simulink subsystem "Day6_Scenario_1"  (R2024a)
settings: Solver=VariableStepAuto  StartTime=0.0  StopTime=10.0  RelTol=1e-3
undefined symbols (not defined in the file): DiscIntNeverNeededParam, route1_waypoint, route2_waypoint, route3_waypoint
libraries: CarMaker4SL x42, simulink x1
(part 2 of 2)

== matlab function Day6_Scenario_1/MATLAB Function19 ==
  settings: sampleTime=0.1
  data: ego_pos input; ego_yaw input; ego_vx input; target_speed input; route1_waypoint input; FrontTireAngle output; DesiredAx output; x_local output; y_local output; lane_id_out output; route2_waypoint input; route3_waypoint input; dt input
% function [FrontTireAngle, DesiredAx, x_local, y_local, lane_id_out] = lane_follower_allin1( ...
%     ego_pos, ego_yaw, ego_vx, target_speed, ...
%     route1_waypoint, route2_waypoint, route3_waypoint, dt)
% % 하나의 블록에서 10초마다 차선 바꾸면서 해당 차선 추종
% 
% %% 1. 10초 주기 lane_id 변경 (시퀀스)
% persistent elapsed lane_idx
% seq = [1 2 3 2 1 2]; % 순환 패턴
% Nseq = length(seq);
% T = 15; % 10초
% 
% if isempty(elapsed)
%     elapsed = 0;
%     lane_idx = 1;
% end
% 
% elapsed = elapsed + dt;
% if elapsed >= T
%     lane_idx = mod(lane_idx, Nseq) + 1;
%     elapsed = 0;
% end
% lane_id = seq(lane_idx);
% lane_id_out = lane_id; % (디버깅/Scope 출력용)
% 
% %% 2. 차선별 route 선택
% if lane_id == 1
%     waypoints = route1_waypoint;
% elseif lane_id == 2
%     waypoints = route2_waypoint;
% elseif lane_id == 3
%     waypoints = route3_waypoint;
% else
%     waypoints = route1_waypoint; % 예외
% end
% 
% %% 3. 이하 기존 웨이포인트 추종 로직 (필요시 복사/수정)
% ego_x = ego_pos(1);
% ego_y = ego_pos(2);
% 
% % 샘플링
% sample_gap = 10;
% x = waypoints(1:sample_gap:end,1);
% y = waypoints(1:sample_gap:end,2);
% 
% % 이상치 필터링
% dx = diff(x); dy = diff(y);
% d = sqrt(dx.^2 + dy.^2);
% thresh = mean(d) + 4*std(d);
% normal_idx = find([true; d < thresh]);
% x_filt = x(normal_idx);
% y_filt = y(normal_idx);
% 
% % 폐곡선 보장
% if norm([x_filt(1), y_filt(1)] - [x_filt(end), y_filt(end)]) > 1e-3
%     x_filt = [x_filt; x_filt(1)];
%     y_filt = [y_filt; y_filt(1)];
% end
% 
% N = length(x_filt);
% 
% % 보간
% interp_ratio = 3;
% max_interp = min(10000, interp_ratio*N);
% t = (1:N)';
% tq = linspace(1, N, max_interp)';
% route_xq = interp1(t, x_filt, tq, 'spline');
% route_yq = interp1(t, y_filt, tq, 'spline');
% Nq = length(route_xq);
% 
% % 윈도우/인덱스 관리
% persistent prev_idx
% if isempty(prev_idx)
%     dist_init = sqrt((route_xq - ego_x).^2 + (route_yq - ego_y).^2);
%     [~, prev_idx] = min(dist_init);
% end
% 
% window_size = 300;
% idx_win = mod((prev_idx-window_size):(prev_idx+window_size)-1, Nq) + 1;
% 
% dx_win = route_xq(idx_win) - ego_x;
% dy_win = route_yq(idx_win) - ego_y;
% x_local_win = dx_win * cos(-ego_yaw) - dy_win * sin(-ego_yaw);
% y_local_win = dx_win * sin(-ego_yaw) + dy_win * cos(-ego_yaw);
% 
% % 진행방향(dot product) 기반 추종점 선택
% Nw = length(idx_win);
% tangent_vecs = zeros(Nw,2);
% for i=1:Nw
%     ip1 = mod(idx_win(i), Nq) + 1;
%     tangent_vecs(i,1) = route_xq(ip1) - route_xq(idx_win(i));
%     tangent_vecs(i,2) = route_yq(ip1) - route_yq(idx_win(i));
% end
% tangent_norm = sqrt(sum(tangent_vecs.^2,2));
% tangent_vecs = tangent_vecs ./ max(tangent_norm, 1e-6);
% 
% ego_heading = [cos(ego_yaw), sin(ego_yaw)];
% dotval = tangent_vecs * ego_heading';
% 
% valid_idx = find(x_local_win > 0 & dotval > 0.0);
% 
% if isempty(valid_idx)
%     [~, idx_sub] = min(sqrt(dx_win.^2 + dy_win.^2));
%     idx_min = idx_win(idx_sub);
%     idx_local = idx_sub;
% else
%     [~, idx_sub] = min(x_local_win(valid_idx).^2 + y_local_win(valid_idx).^2);
%     idx_min = idx_win(valid_idx(idx_sub));
%     idx_local = valid_idx(idx_sub);
% end
% 
% x_local = x_local_win(idx_local);
% y_local = y_local_win(idx_local);
% cte = y_local;
% prev_idx = mod(idx_min - 1, Nq) + 1;
% 
% % 횡방향 PD 제어 (조향)
% persistent prev_e prev_steer
% if isempty(prev_e)
%     prev_e = 0;
% end
% if isempty(prev_steer)
%     prev_steer = 0;
% end
% Kp = 0.2;   
% Kd = 0.01;
% d_e = (cte - prev_e) / dt;
% raw_steer = (Kp * cte + Kd * d_e);
% prev_e = cte;
% 
% % ====== 조향각 제한 ======
% STEER_LIMIT = 1; % [rad], ±28도 정도
% raw_steer = max(min(raw_steer, STEER_LIMIT), -STEER_LIMIT);
% 
% % ====== 조향각 변화율 제한 추가 ======
% MAX_STEER_RATE = 0.03;  % [rad/step] (예: 0.02rad/0.001s → 20rad/s)
% delta_steer = raw_steer - prev_steer;
% delta_steer = max(min(delta_steer, MAX_STEER_RATE), -MAX_STEER_RATE);
% 
% FrontTireAngle = prev_steer + delta_steer;
% prev_steer = FrontTireAngle;
% 
% 
% 
% % 종방향 PID 제어 (속도/가속) 및 속도 리미트
% vel_error = target_speed - ego_vx;
% persistent int_v prev_v
% if isempty(int_v)
%     int_v = 0;
%     prev_v = 0;
% end
% Kp_v = 1.2;
% Ki_v = 0.2;
% Kd_v = 0.05;
% int_v = int_v + vel_error * dt;
% d_v = (vel_error - prev_v) / dt;
% DesiredAx = Kp_v * vel_error + Ki_v * int_v + Kd_v * d_v;
% prev_v = vel_error;
% 
% MAX_SPEED = 15;
% if ego_vx >= MAX_SPEED && target_speed >= MAX_SPEED
%     DesiredAx = min(DesiredAx, 0);
% end
% 
% end



%% 

function [FrontTireAngle, DesiredAx, x_local, y_local, lane_id_out] = lane_follower_allin1( ...
    ego_pos, ego_yaw, ego_vx, target_speed, ...
    route1_waypoint, route2_waypoint, route3_waypoint, dt)
% 하나의 블록에서 10초마다 차선 바꾸면서 해당 차선 추종

%% 1. 10초 주기 lane_id 변경 (시퀀스)
persistent elapsed lane_idx
seq = [1 2 1]; % 순환 패턴
Nseq = length(seq);
T = 15; % 15초

if isempty(elapsed)
    elapsed = 0;
    lane_idx = 1;
end

elapsed = elapsed + dt;
if elapsed >= T
    lane_idx = mod(lane_idx, Nseq) + 1;
    elapsed = 0;
end
lane_id = seq(lane_idx);
lane_id_out = lane_id; % (디버깅/Scope 출력용)

%% 2. 차선별 route 선택
if lane_id == 1
    waypoints = route1_waypoint;
elseif lane_id == 2
    waypoints = route2_waypoint;
elseif lane_id == 3
    waypoints = route3_waypoint;
else
    waypoints = route1_waypoint; % 예외
end

%% 3. 웨이포인트 추종 로직
ego_x = ego_pos(1);
ego_y = ego_pos(2);

% 샘플링
sample_gap = 10;
x = waypoints(1:sample_gap:end,1);
y = waypoints(1:sample_gap:end,2);

% 이상치 필터링
dx = diff(x); dy = diff(y);
d = sqrt(dx.^2 + dy.^2);
thresh = mean(d) + 4*std(d);
normal_idx = find([true; d < thresh]);
x_filt = x(normal_idx);
y_filt = y(normal_idx);

% 폐곡선 보장
if norm([x_filt(1), y_filt(1)] - [x_filt(end), y_filt(end)]) > 1e-3
    x_filt = [x_filt; x_filt(1)];
    y_filt = [y_filt; y_filt(1)];
end

N = length(x_filt);

% 보간
interp_ratio = 3;
max_interp = min(10000, interp_ratio*N);
t = (1:N)';
tq = linspace(1, N, max_interp)';
route_xq = interp1(t, x_filt, tq, 'spline');
route_yq = interp1(t, y_filt, tq, 'spline');
Nq = length(route_xq);

% 윈도우/인덱스 관리
persistent prev_idx
if isempty(prev_idx)
    dist_init = sqrt((route_xq - ego_x).^2 + (route_yq - ego_y).^2);
    [~, prev_idx] = min(dist_init);
end

window_size = 300;
idx_win = mod((prev_idx-window_size):(prev_idx+window_size)-1, Nq) + 1;

dx_win = route_xq(idx_win) - ego_x;
dy_win = route_yq(idx_win) - ego_y;
x_local_win = dx_win * cos(-ego_yaw) - dy_win * sin(-ego_yaw);
y_local_win = dx_win * sin(-ego_yaw) + dy_win * cos(-ego_yaw);

% 진행방향(dot product) 기반 추종점 선택
Nw = length(idx_win);
tangent_vecs = zeros(Nw,2);
for i=1:Nw
    ip1 = mod(idx_win(i), Nq) + 1;
    tangent_vecs(i,1) = route_xq(ip1) - route_xq(idx_win(i));
    tangent_vecs(i,2) = route_yq(ip1) - route_yq(idx_win(i));
end
tangent_norm = sqrt(sum(tangent_vecs.^2,2));
tangent_vecs = tangent_vecs ./ max(tangent_norm, 1e-6);

ego_heading = [cos(ego_yaw), sin(ego_yaw)];
dotval = tangent_vecs * ego_heading';

valid_idx = find(x_local_win > 0 & dotval > 0.0);

if isempty(valid_idx)
    [~, idx_sub] = min(sqrt(dx_win.^2 + dy_win.^2));
    idx_min = idx_win(idx_sub);
    idx_local = idx_sub;
else
    [~, idx_sub] = min(x_local_win(valid_idx).^2 + y_local_win(valid_idx).^2);
    idx_min = idx_win(valid_idx(idx_sub));
    idx_local = valid_idx(idx_sub);
end

x_local = x_local_win(idx_local);
y_local = y_local_win(idx_local);
cte = y_local;
prev_idx = mod(idx_min - 1, Nq) + 1;

% --- 횡방향 PD 제어 (조향) + 제한 ---
persistent prev_e prev_steer
if isempty(prev_e)
    prev_e = 0;
end
if isempty(prev_steer)
    prev_steer = 0;
end
Kp = 0.04;
Kd = 0.04;
d_e = (cte - prev_e) / dt;
raw_steer = (Kp * cte + Kd * d_e);
prev_e = cte;

% 조향각 제한
STEER_LIMIT = 0.7;
raw_steer = max(min(raw_steer, STEER_LIMIT), -STEER_LIMIT);

% 조향각 변화율 제한
MAX_STEER_RATE = 0.015;
delta_steer = raw_steer - prev_steer;
delta_steer = max(min(delta_steer, MAX_STEER_RATE), -MAX_STEER_RATE);
FrontTireAngle = prev_steer + delta_steer;
prev_steer = FrontTireAngle;

% --- 종방향 PID 제어 (속도/가속) ---
vel_error = target_speed - ego_vx;
persistent int_v prev_v
if isempty(int_v)
    int_v = 0;
    prev_v = 0;
end
Kp_v = 1.2;
Ki_v = 0.2;
Kd_v = 0.05;
int_v = int_v + vel_error * dt;
d_v = (vel_error - prev_v) / dt;
DesiredAx = Kp_v * vel_error + Ki_v * int_v + Kd_v * d_v;
prev_v = vel_error;

% --- 자차 속도 제한 ---
MAX_SPEED = 15;
if ego_vx >= MAX_SPEED && target_speed >= MAX_SPEED
    DesiredAx = min(DesiredAx, 0);
end

% --- 조향각에 따라 가속 억제 ---
STEER_THRES = 0.12;  % [rad] (약 7도)
if abs(FrontTireAngle) > STEER_THRES
    DesiredAx = min(DesiredAx, 0);   % 감속 또는 유지만 허용
end

end

== matlab function Day6_Scenario_1/MATLAB Function8 ==
  settings: sampleTime=0.1
  data: ego_pos input; path_keep_local output; ego_yaw input; path_left_local output; path_right_local output
function [path_keep_local, path_left_local, path_right_local] = lane_path_generator(ego_pos, ego_yaw)
%#codegen

% === 1) 전역 기준 중앙 경로 정의 (2차선 중심선) ===
path_keep = [...
     0,   0;
    10,   0;
    20,   0;
    30,   0;
    40,   0;
    50,   0;
    60,   0;
    70,   0;
    80,   0;
    90,   0;
   100,   0];

% === 2) 차선 폭 설정 ===
lane_width = 3.5;

% === 3) 각 차선 경로 생성 (전역 좌표 기준) ===
path_left  = path_keep;
path_right = path_keep;

for i = 1:size(path_keep,1)
    path_left(i,2)  = path_keep(i,2)  - lane_width;  % y축 - 방향 (안쪽)
    path_right(i,2) = path_keep(i,2)  + lane_width;  % y축 + 방향 (바깥쪽)
end

% === 4) 전역 경로 → 차량 기준 로컬 좌표로 변환 ===
path_keep_local  = global_to_local(path_keep,  ego_pos, ego_yaw);
path_left_local  = global_to_local(path_left,  ego_pos, ego_yaw);
path_right_local = global_to_local(path_right, ego_pos, ego_yaw);

end

% === 보조 함수: 전역 → 로컬 변환 ===
function local = global_to_local(global_path, ego_pos, ego_yaw)
N = size(global_path,1);
local = zeros(N,2);

cos_yaw = cos(ego_yaw);
sin_yaw = sin(ego_yaw);

for i = 1:N
    dx = global_path(i,1) - ego_pos(1);
    dy = global_path(i,2) - ego_pos(2);

    % 로컬 좌표 변환: R(-yaw) * [dx; dy]
    x_local =  dx * cos_yaw + dy * sin_yaw;
    y_local = -dx * sin_yaw + dy * cos_yaw;

    local(i,:) = [x_local, y_local];
end
end

== matlab function Day6_Scenario_1/MATLAB Function10 ==
  settings: sampleTime=0.1
  data: ego_pos input; best_path_idx output; traffic0_pos input; traffic1_pos input; traffic2_pos input
function best_path_idx = FSM_Trajectory_planning(ego_pos, traffic0_pos, traffic1_pos, traffic2_pos)
%#codegen

% 안전거리 기준
safe_distance = 15.0;

% === 1) 각 차선별 전방 거리 계산 ===
d_left  = traffic0_pos(1) - ego_pos(1);  % 1차선
d_keep  = traffic1_pos(1) - ego_pos(1);  % 2차선
d_right = traffic2_pos(1) - ego_pos(1);  % 3차선

% === 2) 안전거리 미만은 제외 ===
if d_left < safe_distance
    d_left = -Inf;
end
if d_keep < safe_distance
    d_keep = -Inf;
end
if d_right < safe_distance
    d_right = -Inf;
end

% === 3) 가장 먼 차선 선택 ===
[val, idx] = max([d_keep, d_left, d_right]);  % 1=keep, 2=left, 3=right

% === 4) 출력 ===
best_path_idx = int32(idx);
end

== matlab function Day6_Scenario_1/MATLAB Function11 ==
  settings: sampleTime=0.1
  data: ego_pos input; tire_angle_keep output; path_keep input
function tire_angle_keep = Ego_motion_control(ego_pos, path_keep)
%#codegen

% PID 이득값
Kp = 1.0;
Ki = 0.1;
Kd = 0.5;

% 샘플링 시간
dt = 0.001;

% 이전 상태 저장
persistent int_e prev_e
if isempty(int_e)
    int_e = 0;
    prev_e = 0;
end

% === 1) Cross Track Error 계산 ===
% 기준 경로 중 가장 가까운 점과의 y좌표 오차 사용 (단순한 CTE 추정)
dist = vecnorm(path_keep' - ego_pos);      % 각 포인트까지 거리
[~, min_idx] = min(dist);                  % 가장 가까운 경로점 인덱스
cte = path_keep(min_idx,2);                % y 방향 오차가 CTE (ego는 원점 기준)

% === 2) PID 제어 계산 ===
int_e = int_e + cte * dt;
derivative = (cte - prev_e) / dt;

tire_angle_keep = Kp * cte + Ki * int_e + Kd * derivative;

prev_e = cte;
end

== matlab function Day6_Scenario_1/MATLAB Function12 ==
  settings: sampleTime=0.1
  data: ego_pos input; ego_yaw input; ego_vx input; tire_angle_change output; path_keep input; path_left input; path_right input; traffic0_pos input; traffic1_pos input; traffic2_pos input; best_path_idx input; desired_ax output
function [tire_angle_change, desired_ax] = Trajectory_motion_control( ...
    ego_pos, ego_yaw, ego_vx, ...
    path_keep, path_left, path_right, ...
    traffic0_pos, traffic1_pos, traffic2_pos, ...
    best_path_idx)
%#codegen

% 초기화
tire_angle_change = 0;
desired_ax = 0;

% === 1. 경로 선택 ===
if best_path_idx == 2
    path = path_left;
    traffic_pos = traffic0_pos;
elseif best_path_idx == 3
    path = path_right;
    traffic_pos = traffic2_pos;
else
    path = path_keep;  % fallback
    traffic_pos = traffic1_pos;
end

% === 2. Cross Track Error 계산 (단순 추정) ===
dist = vecnorm(path' - ego_pos);
[~, idx] = min(dist);
cte = path(idx, 2);

% === 3. PID 기반 조향 제어 (초기 구현) ===
Kp = 0.01;
Kd = 0.5;
dt = 0.001;

persistent prev_e
if isempty(prev_e)
    prev_e = 0;
end

derivative = (cte - prev_e) / dt;
tire_angle_change = Kp * cte + Kd * derivative;
prev_e = cte;

% === 4. 단순 ACC (전방 거리 기반 종방향 제어) ===
dx = traffic_pos(1) - ego_pos(1);
target_v = 15.0;
time_gap = 1.5;

if dx > 0
    desired_gap = ego_vx * time_gap + 5.0;
    error_gap = dx - desired_gap;
    K_acc = 0.5;
    desired_ax = K_acc * error_gap;
end



% 최고 속도 제한 (30 km/h = 8.33 m/s)
v_max = 8.33;

if ego_vx >= v_max
    % 현재 속도가 제한보다 크면 감속 유도 또는 가속 차단
    if desired_ax > 0
        desired_ax = 0;  % 더 이상 가속하지 않음
    end
end

end

== matlab function Day6_Scenario_1/MATLAB Function13 ==
  settings: sampleTime=0.1
  data: u1 input; y output; u2 input
function y = longitudinal_speed_pd_controller_(u1, u2)
    y = 0;
end

== matlab function Day6_Scenario_1/MATLAB Function1 ==
  settings: sampleTime=0.1
  data: ego_x input; ego_y input; y output; traffic0 input; traffic1 input; traffic2 input; ego_v input; target_speed input
function y = longitudinal_speed_pd_controller_( ...
    ego_x, ego_y, ...
    traffic0, traffic1, traffic2, ...
    ego_v, target_speed)

    % Mux된 traffic 정보 분리
    tx0 = traffic0(1); ty0 = traffic0(2); vx0 = traffic0(3);
    tx1 = traffic1(1); ty1 = traffic1(2); vx1 = traffic1(3);
    tx2 = traffic2(1); ty2 = traffic2(2); vx2 = traffic2(3);

    % 거리 계산
    d0 = sqrt((tx0 - ego_x)^2 + (ty0 - ego_y)^2);
    d1 = sqrt((tx1 - ego_x)^2 + (ty1 - ego_y)^2);
    d2 = sqrt((tx2 - ego_x)^2 + (ty2 - ego_y)^2);

    % 가장 가까운 차량 선택
    [min_dist, idx] = min([d0, d1, d2]);
    vx_list = [vx0, vx1, vx2];
    target_v = vx_list(idx);

    % 추종 여부 판단
    if min_dist < 25
        v_ref = target_v;
    else
        v_ref = target_speed;
    end

    % PD 제어
    Kp = 0.3;
    Kd = 0.1;

    persistent prev_error
    if isempty(prev_error)
        prev_error = 0;
    end

    dt = 0.01;
    error = v_ref - ego_v;
    d_error = (error - prev_error) / dt;

    y = Kp * error + Kd * d_error;

    % Saturation
    y = max(min(y, 3.0), -5.0);

    prev_error = error;
end

== matlab function Day6_Scenario_1/MATLAB Function2 ==
  settings: sampleTime=0.1
  data: u input; y output
function y = lateral_pid_controller_(u)
% u: CrossTrackError
% y: 앞바퀴 조향각 출력 (rad)

    % 게인 설정
    Kp = 0.5;
    Ki = 0.1;
    Kd = 0.001;

    persistent integral prev_error
    if isempty(integral)
        integral = 0;
        prev_error = 0;
    end

    dt = 0.001;  % 제어 주기

    error = u;
    integral = integral + error * dt;
    derivative = (error - prev_error) / dt;

    % PID 계산
    y = Kp * error + Ki * integral + Kd * derivative;

    % 조향각 제한 (±28.6도 ≈ ±0.5 rad)
    max_steer = 0.5;
    y = max(min(y, max_steer), -max_steer);

    prev_error = error;
end

== matlab function Day6_Scenario_1/MATLAB Function14 ==
  settings: sampleTime=0.1
  data: u input; y output
function y = lateral_pid_controller_(u)
    y = 0;
end

== matlab function Day6_Scenario_1/MATLAB Function15 ==
  settings: sampleTime=0.1
  data: ego_pos input; ego_yaw input; ego_vx input; Front_Tire_Angle output; target_speed input; CrossTrackError input; traffic0_pos input; traffic1_pos input; traffic2_pos input; DesiredAx output; cte output; best_path_idx output; path_keep_local input; path_left_local input; path_right_local input
function [Front_Tire_Angle, DesiredAx, cte, best_path_idx] = ...
         Trajectory_Main_Controller( ...
             ego_pos, ego_yaw, ego_vx, target_speed, CrossTrackError, ...
             traffic0_pos, traffic1_pos, traffic2_pos, ...
             path_keep_local, path_left_local, path_right_local)
%#codegen

% ───── FSM 판단: 경로 선택 (Keep / Left / Right) ─────
safe_distance = 15.0;

% Ego 진행 방향 벡터
heading = [cos(ego_yaw); sin(ego_yaw)];

% 상대 위치 벡터
rel_left  = traffic0_pos - ego_pos;
rel_keep  = traffic1_pos - ego_pos;
rel_right = traffic2_pos - ego_pos;

% 전방 거리 계산 (dot product 방식)
d_left  = dot(heading, rel_left);
d_keep  = dot(heading, rel_keep);
d_right = dot(heading, rel_right);

% 안전거리 미만 시 차선 선택 불가
if d_left < 0 || d_left < safe_distance
    d_left = -Inf;
end
if d_keep < 0 || d_keep < safe_distance
    d_keep = -Inf;
end
if d_right < 0 || d_right < safe_distance
    d_right = -Inf;
end

% 최대 거리인 경로 선택
[~, best_path_idx] = max([d_keep, d_left, d_right]);  % 1=Keep, 2=Left, 3=Right

% ───── 선택한 경로로 Cross Track Error 적용 ─────
cte = CrossTrackError;  % 외부 입력으로 주어짐 (기준 경로 기준)

% ───── 횡방향 조향 제어: PID 제어기 ─────
Kp = 0.1;
Kd = 0.5;
Ki = 0.01;
dt = 0.001;

persistent int_e prev_e
if isempty(int_e)
    int_e = 0;
    prev_e = 0;
end

int_e = int_e + cte * dt;
derivative = (cte - prev_e) / dt;
tire_angle = Kp * cte + Ki * int_e + Kd * derivative;
prev_e = cte;

% ───── 종방향 제어: Keep vs. ACC ─────
speed_limit = 20;  % 최고속도 제한 (m/s)

if best_path_idx == 1
    % Keep 차선: 목표 속도 추종 (PD 제어)
    Kp_speed = 1.5;
    DesiredAx = Kp_speed * (target_speed - ego_vx);

    if ego_vx > speed_limit
        DesiredAx = -1.0;
    end

else
    % 차선 변경: 선행 차량 거리 기반 ACC 제어
    if best_path_idx == 2
        front_car = traffic0_pos;
    else
        front_car = traffic2_pos;
    end

    dx = front_car(1) - ego_pos(1);
    desired_gap = ego_vx * 1.5 + 5.0;
    gap_error = dx - desired_gap;

    K_acc = 0.6;
    DesiredAx = K_acc * gap_error;

    if ego_vx > speed_limit
        DesiredAx = -1.0;
    end
end

% ───── 가속도 Saturation ─────
if DesiredAx > 2.0
    DesiredAx = 2.0;
elseif DesiredAx < -3.0
    DesiredAx = -3.0;
end

% ───── 최종 출력 ─────
Front_Tire_Angle = tire_angle;
end

== matlab function Day6_Scenario_1/MATLAB Function20 ==
  settings: sampleTime=0.1
  data: dt input; lane_id output
function lane_id = lane_change_timer(dt)
    % dt: 샘플링 타임 (예: 0.001)
    persistent elapsed lane_idx
    seq = [1 2 3 2 1 2];
    N = length(seq);
    T = 10; % 10초

    if isempty(elapsed)
        elapsed = 0;
        lane_idx = 1;
    end

    elapsed = elapsed + dt;

    if elapsed >= T
        lane_idx = mod(lane_idx, N) + 1;
        elapsed = 0; % 리셋
    end

    lane_id = seq(lane_idx);
end

== stateflow chart Day6_Scenario_1/Chart ==
  (default) -> (junction 1)
  (junction 1) -> (junction 3) [order 1] : [i<99]
      | {i = i + 1;}
  (junction 1) -> (junction 7) [order 2] : {i=0;}
  (junction 3) -> (junction 5)
  (junction 5) -> (junction 7)
  (junction 7) -> (junction 10)
  (junction 10) -> (junction 12) [order 1] : [rem(i,50) == 0]
      | {do_Logic;}
  (junction 10) -> (junction 18) [order 2]
  (junction 12) -> (junction 16)
  (junction 16) -> (junction 18)
  (junction 18) -> (junction 21)
  (junction 21) -> (junction 34) [order 1] : [rem(i,10000) == 0]
      | {do_10s;}
  (junction 21) -> (junction 32) [order 2]
  (junction 34) -> (junction 31)
  (junction 31) -> (junction 32)
  (junction 32) -> (junction 36)
  data: i local =0
  events: do_Logic output FUNCTION_CALL_EVENT; do_10s output FUNCTION_CALL_EVENT

== matlab function Day6_Scenario_1/MATLAB Function21 ==
  settings: sampleTime=0.1
  data: ego_global input; lead1_global input; lead2_global input; lead3_global input; route1_waypoint input; route2_waypoint input; ego_local_1 output; route3_waypoint input; lead_local_1 output; route1_local output; ego_local_2 output; lead_local_2 output; route2_local output; ego_local_3 output; lead_local_3 output; route3_local output
function [ego_local_1, lead_local_1, route1_local, ...
          ego_local_2, lead_local_2, route2_local, ...
          ego_local_3, lead_local_3, route3_local] = ...
         global_to_local_all(ego_global, lead1_global, lead2_global, lead3_global, ...
                             route1_waypoint, route2_waypoint, route3_waypoint)
% 각 차선별로 Ego/Lead/Waypoints를 해당 차선 기준 로컬로 변환

[ego_local_1, lead_local_1, route1_local] = global_to_local_lane(ego_global, lead1_global, route1_waypoint);
[ego_local_2, lead_local_2, route2_local] = global_to_local_lane(ego_global, lead2_global, route2_waypoint);
[ego_local_3, lead_local_3, route3_local] = global_to_local_lane(ego_global, lead3_global, route3_waypoint);

end

function [ego_local, lead_local, local_wp] = global_to_local_lane(ego_global, lead_global, route_waypoint)
% 해당 차선 기준으로 변환

N = size(route_waypoint,1);

% 1) 웨이포인트 로컬 변환
local_wp = zeros(N,2);
for i = 1:N
    ref = route_waypoint(i,:);
    if i < N
        ref2 = route_waypoint(i+1,:);
    else
        ref2 = route_waypoint(i,:);
    end
    ref_yaw = atan2(ref2(2)-ref(2), ref2(1)-ref(1));
    dx = route_waypoint(i,1) - ref(1);
    dy = route_waypoint(i,2) - ref(2);
    x_local = dx * cos(-ref_yaw) - dy * sin(-ref_yaw);
    y_local = dx * sin(-ref_yaw) + dy * cos(-ref_yaw);
    local_wp(i,:) = [x_local, y_local];
end

% 2) Ego/Lead 글로벌 → 로컬
ego_local = global2local(ego_global, route_waypoint);
lead_local = global2local_lead(lead_global, ego_global, route_waypoint);
end

function local = global2local(ego_global, route_waypoint)
% Ego 글로벌 → 로컬 (차선 기준)
wp = route_waypoint;
ego_x = ego_global(1); ego_y = ego_global(2); ego_yaw = ego_global(3);
dists = sqrt((wp(:,1)-ego_x).^2 + (wp(:,2)-ego_y).^2);
[~, idx] = min(dists);
wp_ref = wp(idx,:);
if idx < size(wp,1)
    ref_x2 = wp(idx+1,1); ref_y2 = wp(idx+1,2);
else
    ref_x2 = wp(idx,1); ref_y2 = wp(idx,2);
end
ref_yaw = atan2(ref_y2-wp_ref(2), ref_x2-wp_ref(1));
dx = ego_x - wp_ref(1);
dy = ego_y - wp_ref(2);
x_local =  dx*cos(-ref_yaw) - dy*sin(-ref_yaw);
y_local =  dx*sin(-ref_yaw) + dy*cos(-ref_yaw);
yaw_local = wrapToPi(ego_yaw - ref_yaw);
local = [x_local; y_local; yaw_local];
end

function lead_local = global2local_lead(lead_global, ego_global, route_waypoint)
% 선행차 글로벌 → 로컬
wp = route_waypoint;
lead_x = lead_global(1); lead_y = lead_global(2);
vx = lead_global(3); vy = lead_global(4);
dists = sqrt((wp(:,1)-lead_x).^2 + (wp(:,2)-lead_y).^2);
[~, idx] = min(dists);
wp_ref = wp(idx,:);
if idx < size(wp,1)
    ref_x2 = wp(idx+1,1); ref_y2 = wp(idx+1,2);
else
    ref_x2 = wp(idx,1); ref_y2 = wp(idx,2);
end
ref_yaw = atan2(ref_y2-wp_ref(2), ref_x2-wp_ref(1));
dx = lead_x - wp_ref(1);
dy = lead_y - wp_ref(2);
x_local =  dx*cos(-ref_yaw) - dy*sin(-ref_yaw);
y_local =  dx*sin(-ref_yaw) + dy*cos(-ref_yaw);
vx_local = vx*cos(-ref_yaw) - vy*sin(-ref_yaw);
vy_local = vx*sin(-ref_yaw) + vy*cos(-ref_yaw);
lead_local = [x_local; y_local; vx_local; vy_local];
end

== matlab function Day6_Scenario_1/MATLAB Function17 ==
  settings: sampleTime=0.1
  data: path_keep_local output; path_left_local output; path_right_local output; ego_pos input; ego_yaw input; route2_waypoint input; route1_waypoint input; route3_waypoint input
function [path_keep_local, path_left_local, path_right_local] = ...
    global_to_local_path(ego_pos, ego_yaw, ...
                         route2_waypoint, route1_waypoint, route3_waypoint)
%#codegen

% 입력이 부족할 경우 방어 처리
if numel(ego_pos) < 2
    ego_pos = [0; 0];  % 기본값 또는 return
end

% 각 경로 변환
path_keep_local  = convert_to_local(route2_waypoint, ego_pos, ego_yaw);
path_left_local  = convert_to_local(route1_waypoint, ego_pos, ego_yaw);
path_right_local = convert_to_local(route3_waypoint, ego_pos, ego_yaw);
end

function local_path = convert_to_local(global_path, ego_pos, ego_yaw)

    if size(global_path, 2) < 2  % y값 존재 여부 확인
        local_path = zeros(1, 2);  % 빈 경로 방지
        return;
    end

    if isrow(ego_pos)
        ego_pos = ego_pos';  % row → column
    end

    N = size(global_path, 1);
    local_path = zeros(N, 2);

    c = cos(ego_yaw);
    s = sin(ego_yaw);

    for i = 1:N
        dx = global_path(i,1) - ego_pos(1);
        dy = global_path(i,2) - ego_pos(2);

        x_local =  dx * c + dy * s;
        y_local = -dx * s + dy * c;

        local_path(i,:) = [x_local, y_local];
    end
end

== matlab function Day6_Scenario_1/MATLAB Function22 ==
  settings: sampleTime=0.1
  data: ego_local_1 input; lead_local_1 input; route1_local input; ego_local_2 input; lane_id output; lead_local_2 input; overtake_flag output; target_local_waypoint output; route2_local input; ego_local_3 input; lead_local_3 input; route3_local input; lane_id_in input; target_ego_local output; target_lead_local output
function [lane_id, overtake_flag, target_local_waypoint, target_ego_local, target_lead_local] = ...
    lane_overtake_fsm(ego_local_1, lead_local_1, route1_local, ...
                      ego_local_2, lead_local_2, route2_local, ...
                      ego_local_3, lead_local_3, route3_local, ...
                      lane_id_in)
% 간단 FSM: 느린차 추월, 기본은 1차선 → 2차선 → 3차선 (예시, 맞춤화 필요)

persistent prev_lane_id overtake_mode
if isempty(prev_lane_id)
    prev_lane_id = lane_id_in;
    overtake_mode = 0; % 0: 평시, 1: 추월중
end

% 추월 조건(예시): 앞차 거리 7m 이하 && 속도 차 0.3m/s 이상 느림
SWITCH_DIST = 7;      % [m]
SPEED_DIFF = 0.3;     % [m/s]

% 현재 차선 정보 선택
switch prev_lane_id
    case 1
        ego = ego_local_1;
        lead = lead_local_1;
        route = route1_local;
        % 선행차와 거리/속도 차
        dx = lead(1) - ego(1);
        rel_v = lead(3) - 0; % lead 속도 - ego(예시, 필요시 ego vx 추가)
        if (dx < SWITCH_DIST) && (rel_v < -SPEED_DIFF)
            overtake_mode = 1;
            lane_id = 2;
        else
            overtake_mode = 0;
            lane_id = 1;
        end
    case 2
        ego = ego_local_2;
        lead = lead_local_2;
        route = route2_local;
        dx = lead(1) - ego(1);
        rel_v = lead(3) - 0;
        % 추월 중 2차선 유지, 임의조건 예시
        if overtake_mode == 1 && (dx > SWITCH_DIST || rel_v > -SPEED_DIFF)
            overtake_mode = 0;
            lane_id = 1; % 추월 끝나면 원복(예시)
        else
            lane_id = 2;
        end
    case 3
        ego = ego_local_3;
        lead = lead_local_3;
        route = route3_local;
        lane_id = 3; % 실제론 3차선 추월 구현 가능, 예시는 1~2만
    otherwise
        ego = ego_local_1;
        lead = lead_local_1;
        route = route1_local;
        lane_id = 1;
end

prev_lane_id = lane_id;

% 출력
target_ego_local = ego;
target_lead_local = lead;
target_local_waypoint = route;
overtake_flag = overtake_mode;
end

== matlab function Day6_Scenario_1/MATLAB Function23 ==
  settings: sampleTime=0.1
  data: ego_local input; lead_local input; local_waypoints input; target_speed input; steering_angle output; desired_ax output
function [steering_angle, desired_ax] = path_tracking_controller(ego_local, lead_local, local_waypoints, target_speed)
% 입력:
%   ego_local:      [x; y; yaw]
%   lead_local:     [x; y; vx; vy]
%   local_waypoints: [N x 2]
%   target_speed:   scalar
% 출력:
%   steering_angle: 조향각 (rad)
%   desired_ax:     종방향 가속도 (m/s^2)

% == 1. 횡방향 제어: Pure Pursuit, Stanley, 혹은 PID (아래는 PID 예시) ==
% 차선 중심까지의 Cross Track Error 계산 (가장 가까운 웨이포인트 기준)
dists = sqrt((local_waypoints(:,1)-ego_local(1)).^2 + (local_waypoints(:,2)-ego_local(2)).^2);
[~, idx] = min(dists);
target_point = local_waypoints(idx,:);
cte = target_point(2);   % y_local이 lateral error로 사용됨 (도로 중심선 기준)

% PID 횡방향 제어
Kp_steer = 2.0;
Ki_steer = 0.0;
Kd_steer = 0.1;

persistent int_e prev_e
dt = 0.001;
if isempty(int_e)
    int_e = 0; prev_e = 0;
end
int_e = int_e + cte*dt;
d_e = (cte - prev_e)/dt;
steering_angle = Kp_steer*cte + Ki_steer*int_e + Kd_steer*d_e;
prev_e = cte;

% == 2. 종방향 제어: ACC (간단히 PID 기반으로) ==
ego_vx = 0; % 로컬 vx가 없는 경우, 속도 센서 등에서 받아야 함 (예: ego_global_vx 등)
if numel(ego_local) >= 4
    ego_vx = ego_local(4);
else
    ego_vx = 0; % 미정의일 경우 0
end

% Lead 차량과의 거리 기반으로 ACC (간단 버전)
lead_dx = lead_local(1) - ego_local(1);   % 전방 거리
desired_gap = 5; % 원하는 안전거리 [m]
gap_error = lead_dx - desired_gap;

Kp_acc = 0.5;
Kd_acc = 0.1;
desired_ax = Kp_acc*(target_speed - ego_vx) + Kd_acc*gap_error;

% Saturation (출력 제한)
max_steer = 0.4; % [rad]
if steering_angle > max_steer
    steering_angle = max_steer;
elseif steering_angle < -max_steer
    steering_angle = -max_steer;
end

max_acc = 2; min_acc = -4;
if desired_ax > max_acc
    desired_ax = max_acc;
elseif desired_ax < min_acc
    desired_ax = min_acc;
end

end

== matlab function Day6_Scenario_1/MATLAB Function4 ==
  settings: sampleTime=0.1
  data: ego_x input; path_keep output; ego_y input; ego_yaw input; path_left output; path_right output
function [path_keep, path_left, path_right] = ...
         TrajectoryGenerator(ego_x, ego_y, ego_yaw)

lane_width = 3.5;
path_length = 30.0;
N = 50;

path_keep  = generate_quintic_path(ego_x, ego_y, ego_yaw, 0.0, path_length, N);
path_left  = generate_quintic_path(ego_x, ego_y, ego_yaw, +lane_width, path_length, N);
path_right = generate_quintic_path(ego_x, ego_y, ego_yaw, -lane_width, path_length, N);

end

function path = generate_quintic_path(x0, y0, yaw0, d_offset, s_total, N)
    % 초기 조건
    s0 = 0; ds0 = 1; dds0 = 0;
    d0 = d_offset; dd0 = 0; ddd0 = 0;

    % 최종 조건
    sf = s_total;
    dsf = 1; ddsf = 0;
    df = d_offset; ddf = 0; dddf = 0;

    % s 값 생성
    s = linspace(s0, sf, N);

    % 다항식 계수 행렬
    A = [1 s0 s0^2 s0^3 s0^4 s0^5;
         0 1  2*s0  3*s0^2 4*s0^3 5*s0^4;
         0 0  2     6*s0   12*s0^2 20*s0^3;
         1 sf sf^2 sf^3 sf^4 sf^5;
         0 1  2*sf  3*sf^2 4*sf^3 5*sf^4;
         0 0  2     6*sf   12*sf^2 20*sf^3];

    b = [d0; dd0; ddd0; df; ddf; dddf];

    coeff = A \ b;

    % 궤적 계산
    d = polyval(flip(coeff'), s);

    x_local = s;
    y_local = d;

    % 회전 + 위치 이동 (로컬 → 글로벌)
    cos_yaw = cos(yaw0);
    sin_yaw = sin(yaw0);
    x_global = x0 + x_local * cos_yaw - y_local * sin_yaw;
    y_global = y0 + x_local * sin_yaw + y_local * cos_yaw;

    path = [x_global', y_global'];
end

== matlab function Day6_Scenario_1/MATLAB Function3 ==
  settings: sampleTime=0.1
  data: path_keep input; path_left input; path_right input; best_path_idx input; steer output; ego_x input; ego_y input; ego_yaw input; t0_x input; t0_y input; t0_vx input; t1_x input; t1_y input; t1_vx input; t2_x input; t2_y input; t2_vx input; ego_vx input; target_speed input; accel output; overtake_flag output
function [steer, accel, overtake_flag]  = lateral_pid_controller_( ...
    path_keep, path_left, path_right, ...
    best_path_idx, ...
    ego_x, ego_y, ego_yaw, ...
    t0_x, t0_y, t0_vx, ...
    t1_x, t1_y, t1_vx, ...
    t2_x, t2_y, t2_vx, ...
    ego_vx, ...
    target_speed)

% ────────────── 설정값 ──────────────
Kp_lat = 2.0;
Ki_lat = 0.5;
Kd_lat = 1;
dt     = 0.001;
steer_max = 0.26;  % 약 ±15도 (rad)

% ────────────── 초기 2초는 경로 변경 금지 ──────────────
persistent time_acc
if isempty(time_acc)
    time_acc = 0;
end
time_acc = time_acc + dt;

if time_acc < 2.0
    best_path_idx = 1;
end

% ────────────── 경로 선택 및 유효성 확인 ──────────────
if best_path_idx == 1 && size(path_keep,2) >= 2
    path = path_keep;
elseif best_path_idx == 2 && size(path_left,2) >= 2
    path = path_left;
elseif best_path_idx == 3 && size(path_right,2) >= 2
    path = path_right;
else
    path = zeros(50,2);  % fallback: 빈 경로 방지
end

% ────────────── CTE 계산 (로컬 기준, yaw 반영) ──────────────
dx = path(:,1) - ego_x;
dy = path(:,2) - ego_y;
dists = sqrt(dx.^2 + dy.^2);
[~, idx_min] = min(dists);

cos_yaw = cos(ego_yaw);
sin_yaw = sin(ego_yaw);
x_local =  cos_yaw * dx(idx_min) + sin_yaw * dy(idx_min);
y_local = -sin_yaw * dx(idx_min) + cos_yaw * dy(idx_min);
cte = y_local;

% ────────────── 횡방향 제어 (조향각) ──────────────
persistent int_e_lat prev_e_lat
if isempty(int_e_lat)
    int_e_lat = 0;
    prev_e_lat = 0;
end

if abs(cte) > 0.5
    int_e_lat = int_e_lat + cte * dt;
    d_e = (cte - prev_e_lat) / dt;
    steer = Kp_lat * cte + Ki_lat * int_e_lat + Kd_lat * d_e;
    steer = -steer;
    steer = max(min(steer, steer_max), -steer_max);  % 제한
else
    steer = 0;
end
prev_e_lat = cte;

% ────────────── 종방향 제어 (가장 가까운 차량 추종) ──────────────
d0 = sqrt((t0_x - ego_x)^2 + (t0_y - ego_y)^2);
d1 = sqrt((t1_x - ego_x)^2 + (t1_y - ego_y)^2);
d2 = sqrt((t2_x - ego_x)^2 + (t2_y - ego_y)^2);

[min_dist, idx_d] = min([d0, d1, d2]);
vx_list = [t0_vx, t1_vx, t2_vx];
target_v = vx_list(idx_d);

% 추월 조건: 가까우면서 ego가 더 빠를 때
if min_dist < 25 && ego_vx > target_v
    v_ref = target_v;
    overtake_flag = 1;
else
    v_ref = target_speed;
    overtake_flag = 0;
end

% ────────────── 종방향 가속도 PID 제어 ──────────────
Kp_long = 3;
Kd_long = 0.5;

persistent prev_err_long
if isempty(prev_err_long)
    prev_err_long = 0;
end

err_long = v_ref - ego_vx;
derr_long = (err_long - prev_err_long) / dt;
accel = Kp_long * err_long + Kd_long * derr_long;
accel = max(min(accel, 3.0), -5.0);
prev_err_long = err_long;

% ────────────── 출력 크기 명시 (Simulink 안전용) ──────────────
steer = double(steer);
accel = double(accel);
overtake_flag = double(overtake_flag);

end

== matlab function Day6_Scenario_1/MATLAB Function5 ==
  settings: sampleTime=0.1
  data: path_keep input; best_path_idx output; path_left input; path_right input; ego_vx input; traffic0 input; traffic1 input; traffic2 input
function best_path_idx = TrajectoryEvaluator( ...
    path_keep, path_left, path_right, ...
    ego_vx, ...
    traffic0, traffic1, traffic2)

% ========================
% 🔧 설정값
% ========================
THRESH_COLLISION = 5.0;         
COST_COLLISION   = 1000;        
COST_LANE_CHANGE = 10;          
T = 2.0;                        

% ========================
% 경로 리스트 구성
% ========================
paths = {path_keep, path_left, path_right};
num_paths = 3;
costs = zeros(1, num_paths);

% ========================
% 비용 계산 루프
% ========================
for i = 1:num_paths
    path = paths{i};

    % --- 선행 차량 예측 (CV 기반, Mux 입력에 맞게)
    pred0 = predict_traffic(traffic0, T);
    pred1 = predict_traffic(traffic1, T);
    pred2 = predict_traffic(traffic2, T);

    % --- 충돌 여부 평가
    collision_cost = 0;
    if check_collision(path, pred0, THRESH_COLLISION)
        collision_cost = collision_cost + COST_COLLISION;
    end
    if check_collision(path, pred1, THRESH_COLLISION)
        collision_cost = collision_cost + COST_COLLISION;
    end
    if check_collision(path, pred2, THRESH_COLLISION)
        collision_cost = collision_cost + COST_COLLISION;
    end

    % --- 차선 변경 penalty
    lane_change_penalty = 0;
    if i ~= 1
        lane_change_penalty = COST_LANE_CHANGE;
    end

    % --- 총 비용 계산
    costs(i) = collision_cost + lane_change_penalty;
end

% ========================
% 최소 비용 경로 선택
% ========================
[~, best_path_idx] = min(costs);

end


function pos_pred = predict_traffic(traffic_vec, T)

% traffic_vec: [8x1] Mux 벡터
% 순서: [x; y; vx; vy; ax; ay; yaw; yawrate]

x  = traffic_vec(1);
y  = traffic_vec(2);
vx = traffic_vec(3);
vy = traffic_vec(4);

x_pred = x + vx * T;
y_pred = y + vy * T;

pos_pred = [x_pred, y_pred];

end


function collision = check_collision(path, obj_pos, threshold)

diffs = path - obj_pos;
dists = sqrt(sum(diffs.^2, 2));
min_dist = min(dists);

collision = (min_dist < threshold);

end
